simulink model "roll_maneuver"  (R2021a)
settings: Solver=VariableStepAuto  StartTime=0.0  StopTime=Torb  RelTol=1e-3
libraries: sharedtransform x2
settings Model: Creator=Laura  LastModifiedBy=Laura

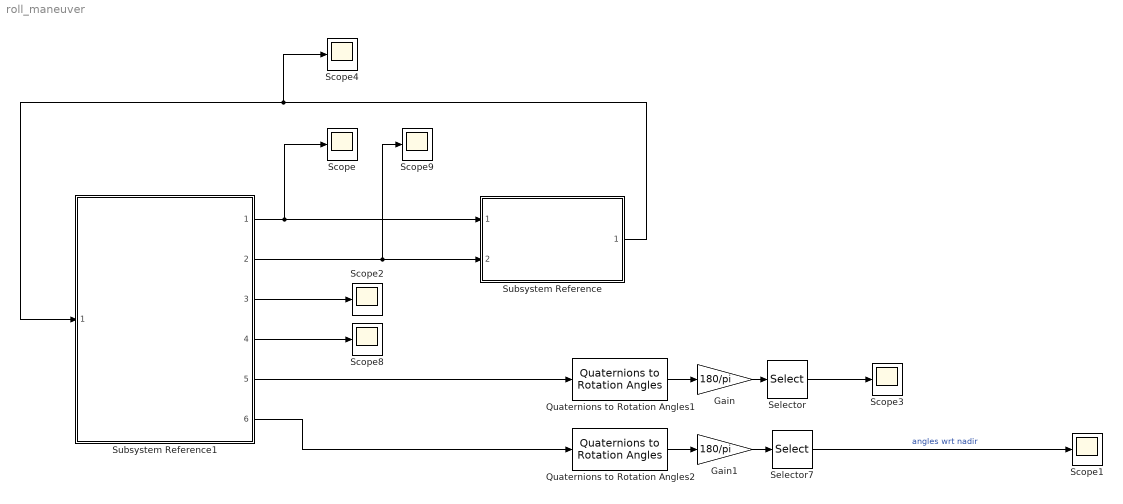
== system roll_maneuver ==
  Gain : Gain  Gain=180/pi
  Gain1 : Gain  Gain=180/pi
  Quaternions to Rotation Angles1 : sharedtransform/Quaternions to Rotation Angles  rotationOrder=ZYX  aMode=aMode
      settings: SourceProductBaseCode=AE,PW,DR,MT,UV,VE
  Quaternions to Rotation Angles2 : sharedtransform/Quaternions to Rotation Angles  rotationOrder=ZYX  aMode=aMode
      settings: SourceProductBaseCode=AE,PW,DR,MT,UV,VE
  Scope{,1..4,8..9} (7 alike) : Scope
  Selector : Selector  InputPortWidth=3  IndexOptions=Index vector (dialog)  Indices=[3 2 1]  OutputSizes=1
  Selector7 : Selector  InputPortWidth=3  IndexOptions=Index vector (dialog)  Indices=[3 2 1]  OutputSizes=1
  Subsystem Reference : Subsystem  ReferencedSubsystem=PD_roll
  Subsystem Reference1 : Subsystem  ReferencedSubsystem=DKE_detumbling
  wires:
  Subsystem Reference1/6 -> Quaternions to Rotation Angles2/1
  Quaternions to Rotation Angles1/1 -> Gain/1
  Subsystem Reference1/5 -> Quaternions to Rotation Angles1/1
  Gain1/1 -> Selector7/1
  Quaternions to Rotation Angles2/1 -> Gain1/1
  Subsystem Reference1/1 -> Scope/1, Subsystem Reference/1
  Subsystem Reference1/3 -> Scope2/1
  Subsystem Reference1/4 -> Scope8/1
  Subsystem Reference1/2 -> Scope9/1, Subsystem Reference/2
  Subsystem Reference/1 -> Scope4/1, Subsystem Reference1/1
  Gain/1 -> Selector/1
  Selector/1 -> Scope3/1
  Selector7/1 -> Scope1/1  "angles wrt nadir"
